simulink model "Super2Out"  (Simulink 6.0)
settings: Solver=ode45  StartTime=0.0  StopTime=10.0  RelTol=1e-3
settings Model: Creator=scaife  LastModifiedBy=scaife  ExtModeAutoUpdateStatusClock=off
settings DataIOCC: SignalLoggingName=sigsOut
settings DebuggingCC: SolverPrmCheckMsg=none
settings HardwareCC: TargetUnknown=on
settings GRTTargetCC: ModelReferenceCompliant=off  MatFileLogging=off

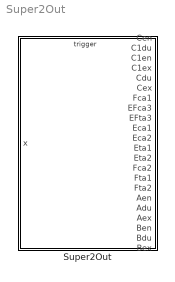
== system Super2Out ==
  Super2Out : Stateflow chart

== stateflow chart Super2Out ==
  state A/
    en: Aen++;
    du: Adu++;
    ex: Aex++;
  state B/
    en: Ben++;
    du: Bdu++;
    ex: Bex++;
  state C/
    en: Cen++;
    du: Cdu++;
    ex: Cex++;
    state C1/
      en: C1en++;
      du: C1du++;
      ex: C1ex++;
    (default) -> C1
  A -> C1 : E
      | {Eca1++;}
      | /Eta1++;
  C1 -> B : E
      | {Eca2++;}
      | /Eta2++;
  (default) -> A
  A -> C : F
      | {Fca1++;}
      | /Fta1++;
  C -> B : F
      | {Fca2++;}
      | /Fta2++;
  B -> A : E||F{EFca3++;}/EFta3++;
  data: x input int32; Cen output int32; C1du output int32; C1en output int32; C1ex output int32; Cdu output int32; Cex output int32; Fca1 output int32; EFca3 output int32; EFta3 output int32; Eca1 output int32; Eca2 output int32; Eta1 output int32; Eta2 output int32; Fca2 output int32; Fta1 output int32; Fta2 output int32; Aen output double; Adu output double; Aex output double; Ben output double; Bdu output double; Bex output double
  events: E input EITHER_EDGE_EVENT; F input EITHER_EDGE_EVENT; G input EITHER_EDGE_EVENT
